simulink model "ESP32Arm6DOF"  (R2024a)
settings: Solver=VariableStepAuto  StartTime=0.0  StopTime=inf  RelTol=1e-3
libraries: arduinolib x7, slpidlib x7, SignalEditorBlockLib x6, arduinosensorlib x2, aerolibanimutils x1
settings Model: Creator=Akbar  LastModifiedBy=Akbar

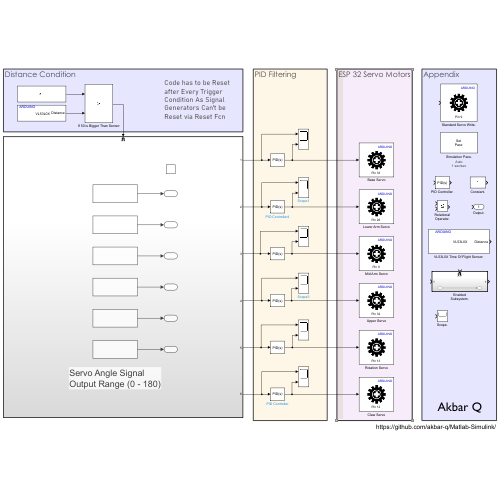
[thumbnail: Simulink's stored preview of the top-level diagram]
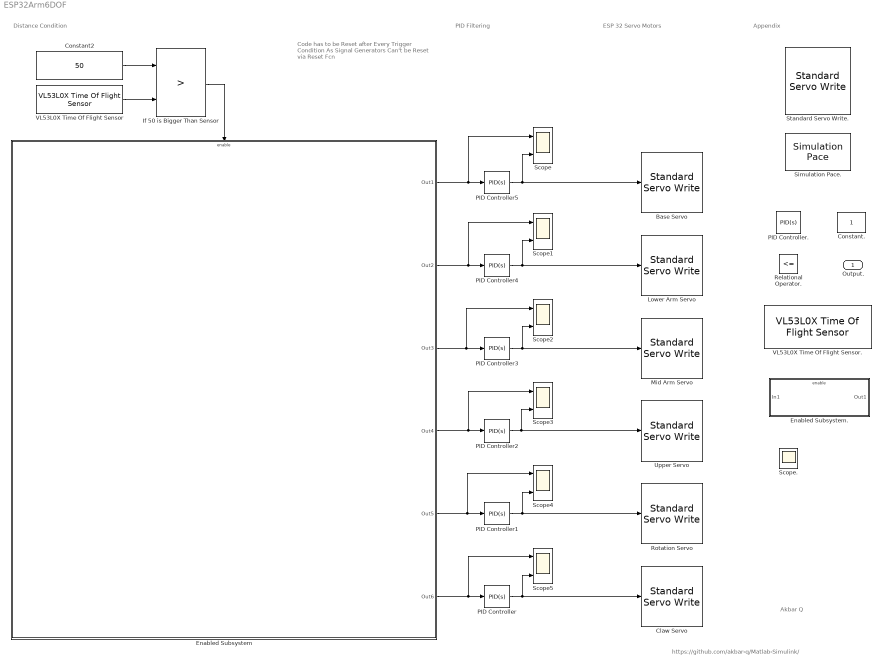
== system ESP32Arm6DOF ==
  note: https://github.com/akbar-q/Matlab-Simulink/
  note: Akbar Q
  note: Code has to be Reset after Every Trigger Condition As Signal Generators Can't be Reset via Reset Fcn
  note: Distance Condition
  note: ESP 32 Servo Motors
  note: PID Filtering
  note: Appendix
  Base Servo : arduinolib/Standard Servo Write  pinNumber=33  ServoIndex=0  blockPlatform=ARDUINO
  Claw Servo : arduinolib/Standard Servo Write  pinNumber=12  ServoIndex=0  blockPlatform=ARDUINO
  Constant. : Constant
  Constant2 : Constant  Value=50
  Enabled Subsystem : Subsystem  TreatAsAtomicUnit=on
  Enabled Subsystem. : Subsystem  TreatAsAtomicUnit=on
  If 50 is Bigger Than Sensor : RelationalOperator  Operator=>  OutDataTypeStr=boolean  RndMeth=Simplest  InputSameDT=off
  Lower Arm Servo : arduinolib/Standard Servo Write  pinNumber=26  ServoIndex=0  blockPlatform=ARDUINO
  Mid Arm Servo : arduinolib/Standard Servo Write  pinNumber=9  ServoIndex=0  blockPlatform=ARDUINO
  PID Controller{,1..5} (6 alike) : slpidlib/PID Controller  Controller=PID  Form=Parallel  TimeDomain=Continuous-time  UseExternalTs=off  SampleTime=-1  IntegratorMethod=Forward Euler  FilterMethod=Forward Euler  ControllerParametersSource=internal  P=1  I=1  UseKiTs=off  D=0  UseExternalDerivativeSource=off  N=100  UseFilter=on  TunerSelectOption=Transfer Function Based (PID Tuner App)  InitialConditionSource=internal  InitialConditionForIntegrator=0  InitialConditionForFilter=0  DifferentiatorICPrevScaledInput=0  ExternalReset=none  TrackingMode=off  Kt=1  LimitOutput=off  SatLimitsSource=internal  UpperSaturationLimit=inf  LowerSaturationLimit=-inf  LinearizeAsGain=on  AntiWindupMode=none  Kb=1  LimitIntegrator=off  UpperIntegratorSaturationLimit=inf  LowerIntegratorSaturationLimit=-inf  POutMin=[]  POutMax=[]  IOutMin=[]  IOutMax=[]  DOutMin=[]  DOutMax=[]  NOutMin=[]  NOutMax=[]  SumOutMin=[]  SumOutMax=[]  SaturationOutMin=[]  SaturationOutMax=[]  PParamMin=[]  PParamMax=[]  IParamMin=[]  IParamMax=[]  DParamMin=[]  DParamMax=[]  NParamMin=[]  NParamMax=[]  KbParamMin=[]  KbParamMax=[]  KtParamMin=[]  KtParamMax=[]  KbOutMin=[]  KbOutMax=[]  KtOutMin=[]  KtOutMax=[]  IntegratorOutMin=[]  IntegratorOutMax=[]  FilterOutMin=[]  FilterOutMax=[]  SumI1OutMin=[]  SumI1OutMax=[]  SumI2OutMin=[]  SumI2OutMax=[]  SumI3OutMin=[]  SumI3OutMax=[]  SumI4OutMin=[]  SumI4OutMax=[]  SumDOutMin=[]  SumDOutMax=[]  DifferentiatorOutMin=[]  DifferentiatorOutMax=[]  FilterDiffOutCoefMin=[]  FilterDiffOutCoefMax=[]  ReciprocalOutMin=[]  ReciprocalOutMax=[]  SumDenOutMin=[]  SumDenOutMax=[]  SumNumOutMin=[]  SumNumOutMax=[]  DivideOutMin=[]  DivideOutMax=[]  UdiffTsProdOutMin=[]  UdiffTsProdOutMax=[]  NTsProdOutMin=[]  NTsProdOutMax=[]  UintegralTsProdOutMin=[]  UintegralTsProdOutMax=[]  UngainTsProdOutMin=[]  UngainTsProdOutMax=[]  ClampingZeroOutDataTypeStr=Inherit: Inherit via back propagation  ClampingZeroOutMin=[]  ClampingZeroOutMax=[]  FilterDenConstantOutDataTypeStr=Inherit: Inherit via back propagation  FilterDenConstantOutMin=[]  FilterDenConstantOutMax=[]  PCopyOutDataTypeStr=Inherit: Inherit via back propagation  PCopyOutMin=[]  PCopyOutMax=[]  NCopyOutDataTypeStr=Inherit: Inherit via back propagation  NCopyOutMin=[]  NCopyOutMax=[]  IntegratorContinuousStateAttributes=''  IntegratorStateMustResolveToSignalObject=off  IntegratorRTWStateStorageClass=Auto  FilterContinuousStateAttributes=''  FilterStateMustResolveToSignalObject=off  FilterRTWStateStorageClass=Auto  ParallelPVariant=InternalParameters  IdealPVariant=Disabled  IVariant=InternalParameters  DVariant=InternalParameters  IntegratorVariant=Continuous  SatVariant=Disabled  AWVariant=Passthrough  PCopyVariant=Disabled  TRVariant=Disabled  FdbkBlocksVariant=Forward  IdealPFdbkVariant=Disabled  SatFdbkVariant=Disabled  DerivativeFilterVariant=ContFilter  NVariant=InternalParameters  NCopyVariant=Disabled  FilterICVariant=InternalICsFilter  IntegratorICVariant=InternalICs  ExternalResetVariant=Disabled  TRSumVariant=Passthrough  SumFdbkVariant=Disabled  SumVariant=Sum_PID  TsampFilterVariant=InternalTs  TsampNgainVariant=Passthrough  TsampIntegralVariant=Disabled_SignalSpec  ExternalSaturationOutDataTypeStr=Inherit: Same as second input  DerivativeSourceVariant=ErrorSignal
  PID Controller. : slpidlib/PID Controller  Controller=PID  Form=Parallel  TimeDomain=Continuous-time  UseExternalTs=off  SampleTime=-1  IntegratorMethod=Forward Euler  FilterMethod=Forward Euler  ControllerParametersSource=internal  P=1  I=1  UseKiTs=off  D=0  UseExternalDerivativeSource=off  N=100  UseFilter=on  TunerSelectOption=Transfer Function Based (PID Tuner App)  InitialConditionSource=internal  InitialConditionForIntegrator=0  InitialConditionForFilter=0  DifferentiatorICPrevScaledInput=0  ExternalReset=none  TrackingMode=off  Kt=1  LimitOutput=off  SatLimitsSource=internal  UpperSaturationLimit=inf  LowerSaturationLimit=-inf  LinearizeAsGain=on  AntiWindupMode=none  Kb=1  LimitIntegrator=off  UpperIntegratorSaturationLimit=inf  LowerIntegratorSaturationLimit=-inf  POutMin=[]  POutMax=[]  IOutMin=[]  IOutMax=[]  DOutMin=[]  DOutMax=[]  NOutMin=[]  NOutMax=[]  SumOutMin=[]  SumOutMax=[]  SaturationOutMin=[]  SaturationOutMax=[]  PParamMin=[]  PParamMax=[]  IParamMin=[]  IParamMax=[]  DParamMin=[]  DParamMax=[]  NParamMin=[]  NParamMax=[]  KbParamMin=[]  KbParamMax=[]  KtParamMin=[]  KtParamMax=[]  KbOutMin=[]  KbOutMax=[]  KtOutMin=[]  KtOutMax=[]  IntegratorOutMin=[]  IntegratorOutMax=[]  FilterOutMin=[]  FilterOutMax=[]  SumI1OutMin=[]  SumI1OutMax=[]  SumI2OutMin=[]  SumI2OutMax=[]  SumI3OutMin=[]  SumI3OutMax=[]  SumI4OutMin=[]  SumI4OutMax=[]  SumDOutMin=[]  SumDOutMax=[]  DifferentiatorOutMin=[]  DifferentiatorOutMax=[]  FilterDiffOutCoefMin=[]  FilterDiffOutCoefMax=[]  ReciprocalOutMin=[]  ReciprocalOutMax=[]  SumDenOutMin=[]  SumDenOutMax=[]  SumNumOutMin=[]  SumNumOutMax=[]  DivideOutMin=[]  DivideOutMax=[]  UdiffTsProdOutMin=[]  UdiffTsProdOutMax=[]  NTsProdOutMin=[]  NTsProdOutMax=[]  UintegralTsProdOutMin=[]  UintegralTsProdOutMax=[]  UngainTsProdOutMin=[]  UngainTsProdOutMax=[]  ClampingZeroOutDataTypeStr=Inherit: Inherit via back propagation  ClampingZeroOutMin=[]  ClampingZeroOutMax=[]  FilterDenConstantOutDataTypeStr=Inherit: Inherit via back propagation  FilterDenConstantOutMin=[]  FilterDenConstantOutMax=[]  PCopyOutDataTypeStr=Inherit: Inherit via back propagation  PCopyOutMin=[]  PCopyOutMax=[]  NCopyOutDataTypeStr=Inherit: Inherit via back propagation  NCopyOutMin=[]  NCopyOutMax=[]  IntegratorContinuousStateAttributes=''  IntegratorStateMustResolveToSignalObject=off  IntegratorRTWStateStorageClass=Auto  FilterContinuousStateAttributes=''  FilterStateMustResolveToSignalObject=off  FilterRTWStateStorageClass=Auto  ParallelPVariant=InternalParameters  IdealPVariant=Disabled  IVariant=InternalParameters  DVariant=InternalParameters  IntegratorVariant=Continuous  SatVariant=Disabled  AWVariant=Passthrough  PCopyVariant=Disabled  TRVariant=Disabled  FdbkBlocksVariant=Forward  IdealPFdbkVariant=Disabled  SatFdbkVariant=Disabled  DerivativeFilterVariant=ContFilter  NVariant=InternalParameters  NCopyVariant=Disabled  FilterICVariant=InternalICsFilter  IntegratorICVariant=InternalICs  ExternalResetVariant=Disabled  TRSumVariant=Passthrough  SumFdbkVariant=Disabled  SumVariant=Sum_PID  TsampFilterVariant=InternalTs  TsampNgainVariant=Passthrough  TsampIntegralVariant=Disabled_SignalSpec  ExternalSaturationOutDataTypeStr=Inherit: Same as second input  DerivativeSourceVariant=ErrorSignal
  Relational Operator. : RelationalOperator  Operator=<=  OutDataTypeStr=boolean  RndMeth=Simplest  InputSameDT=off
  Rotation Servo : arduinolib/Standard Servo Write  pinNumber=13  ServoIndex=0  blockPlatform=ARDUINO
  Scope{,1..5} (6 alike) : Scope  NumInputPorts=2
  Scope. : Scope
  Simulation Pace. : aerolibanimutils/Simulation Pace  SimulationPace=1  SleepMode=Auto  OutputPaceError=off  SampleTime=1/30
  Standard Servo Write. : arduinolib/Standard Servo Write  pinNumber=9  ServoIndex=0  blockPlatform=ARDUINO
  Upper Servo : arduinolib/Standard Servo Write  pinNumber=32  ServoIndex=0  blockPlatform=ARDUINO
  VL53L0X Time Of Flight Sensor : arduinosensorlib/VL53L0X Time Of Flight Sensor  I2CModule=0  I2CAddress=0x29  BitRate=1000000  RangingMode=Default  SampleTime=-1
  VL53L0X Time Of Flight Sensor. : arduinosensorlib/VL53L0X Time Of Flight Sensor  I2CModule=0  I2CAddress=0x29  BitRate=1000000  RangingMode=Default  SampleTime=-1
  Output. : Outport
  wires:
  VL53L0X Time Of Flight Sensor/1 -> If 50 is Bigger Than Sensor/2
  Constant2/1 -> If 50 is Bigger Than Sensor/1
  If 50 is Bigger Than Sensor/1 -> Enabled Subsystem/Enable
  Enabled Subsystem/6(Out6) -> Scope5/1, PID Controller/1
  Enabled Subsystem/5(Out5) -> Scope4/1, PID Controller1/1
  PID Controller/1 -> Scope5/2, Claw Servo/1
  PID Controller1/1 -> Scope4/2, Rotation Servo/1
  PID Controller2/1 -> Upper Servo/1, Scope3/2
  Enabled Subsystem/4(Out4) -> Scope3/1, PID Controller2/1
  PID Controller3/1 -> Scope2/2, Mid Arm Servo/1
  Enabled Subsystem/3(Out3) -> Scope2/1, PID Controller3/1
  PID Controller4/1 -> Scope1/2, Lower Arm Servo/1
  Enabled Subsystem/2(Out2) -> Scope1/1, PID Controller4/1
  Enabled Subsystem/1(Out1) -> Scope/1, PID Controller5/1
  PID Controller5/1 -> Scope/2, Base Servo/1

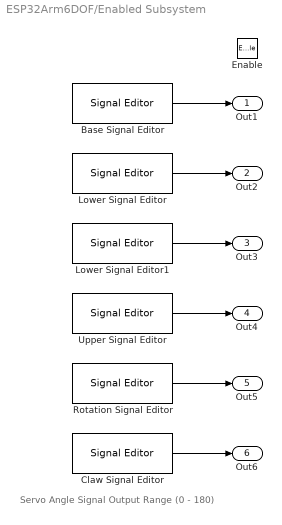
== system ESP32Arm6DOF/Enabled Subsystem ==
  note: Servo Angle Signal
      | Output Range (0 - 180)
  Enable : EnablePort
  Base Signal Editor : SignalEditorBlockLib/Signal Editor  FileName=K:\I-Drive Sync\Cloud-Drive_maa32ocd@bolton.ac.uk\Hobby Projects\GitHub Repos\Matlab-Simulink\ESP32-Arm-5DOF-Interfacing\Path Plans\BasePath.mat  ActiveScenario=Study1  ActiveSignal=BaseSig  IsBus=off  OutputBusObjectStr=Bus: BusObject  SampleTime=0  Interpolate=off  ZeroCross=off  OutputAfterFinalValue=Setting to zero  Unit=inherit  PreserveSignalName=on  ApplySigPropsToAllScenarios=on  ApplySigPropsToAllSignals=off
  Claw Signal Editor : SignalEditorBlockLib/Signal Editor  FileName=K:\I-Drive Sync\Cloud-Drive_maa32ocd@bolton.ac.uk\Hobby Projects\GitHub Repos\Matlab-Simulink\ESP32-Arm-5DOF-Interfacing\Path Plans\ClawPath.mat  ActiveScenario=Study1  ActiveSignal=ClawSignal  IsBus=off  OutputBusObjectStr=Bus: BusObject  SampleTime=0  Interpolate=off  ZeroCross=off  OutputAfterFinalValue=Setting to zero  Unit=inherit  PreserveSignalName=on  ApplySigPropsToAllScenarios=on  ApplySigPropsToAllSignals=off
  Lower Signal Editor : SignalEditorBlockLib/Signal Editor  FileName=K:\I-Drive Sync\Cloud-Drive_maa32ocd@bolton.ac.uk\Hobby Projects\GitHub Repos\Matlab-Simulink\ESP32-Arm-5DOF-Interfacing\Path Plans\LowerPath.mat  ActiveScenario=Study1  ActiveSignal=LowerSignal  IsBus=off  OutputBusObjectStr=Bus: BusObject  SampleTime=0  Interpolate=off  ZeroCross=off  OutputAfterFinalValue=Setting to zero  Unit=inherit  PreserveSignalName=on  ApplySigPropsToAllScenarios=on  ApplySigPropsToAllSignals=off
  Lower Signal Editor1 : SignalEditorBlockLib/Signal Editor  FileName=C:\Users\Akbar\Cloud-Drive_maa32ocd@bolton.ac.uk\Hobby Projects\GitHub Repos\Matlab-Simulink\ESP32-Arm-5DOF-180Servo\Path Plans\MidPath.mat  ActiveScenario=Study1  ActiveSignal=LowerSignal  IsBus=off  OutputBusObjectStr=Bus: BusObject  SampleTime=0  Interpolate=off  ZeroCross=off  OutputAfterFinalValue=Setting to zero  Unit=inherit  PreserveSignalName=on  ApplySigPropsToAllScenarios=on  ApplySigPropsToAllSignals=off
  Rotation Signal Editor : SignalEditorBlockLib/Signal Editor  FileName=K:\I-Drive Sync\Cloud-Drive_maa32ocd@bolton.ac.uk\Hobby Projects\GitHub Repos\Matlab-Simulink\ESP32-Arm-5DOF-Interfacing\Path Plans\RotationPath.mat  ActiveScenario=Study1  ActiveSignal=RotationSignal  IsBus=off  OutputBusObjectStr=Bus: BusObject  SampleTime=0  Interpolate=off  ZeroCross=off  OutputAfterFinalValue=Setting to zero  Unit=inherit  PreserveSignalName=on  ApplySigPropsToAllScenarios=on  ApplySigPropsToAllSignals=off
  Upper Signal Editor : SignalEditorBlockLib/Signal Editor  FileName=K:\I-Drive Sync\Cloud-Drive_maa32ocd@bolton.ac.uk\Hobby Projects\GitHub Repos\Matlab-Simulink\ESP32-Arm-5DOF-Interfacing\Path Plans\UpperPath.mat  ActiveScenario=Study1  ActiveSignal=UpperSignal  IsBus=off  OutputBusObjectStr=Bus: BusObject  SampleTime=0  Interpolate=off  ZeroCross=off  OutputAfterFinalValue=Setting to zero  Unit=inherit  PreserveSignalName=on  ApplySigPropsToAllScenarios=on  ApplySigPropsToAllSignals=off
  Out1 : Outport
  Out2 : Outport  Port=2
  Out3 : Outport  Port=3
  Out4 : Outport  Port=4
  Out5 : Outport  Port=5
  Out6 : Outport  Port=6
  wires:
  Base Signal Editor/1 -> Out1/1
  Lower Signal Editor/1 -> Out2/1
  Upper Signal Editor/1 -> Out4/1
  Rotation Signal Editor/1 -> Out5/1
  Claw Signal Editor/1 -> Out6/1
  Lower Signal Editor1/1 -> Out3/1

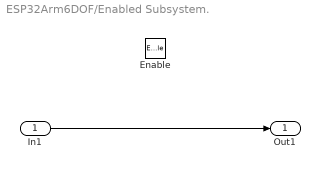
== system ESP32Arm6DOF/Enabled Subsystem. ==
  In1 : Inport
  Enable : EnablePort
  Out1 : Outport
  wires:
  In1/1 -> Out1/1
